simulink library "halin"  (R2021b)
settings: Solver=VariableStepAuto  StartTime=0.0  StopTime=10.0  RelTol=1e-3
undefined symbols (not defined in the file): TRUE
libraries: FVT_lib x100, hcu_lib x41
(part 7 of 10)

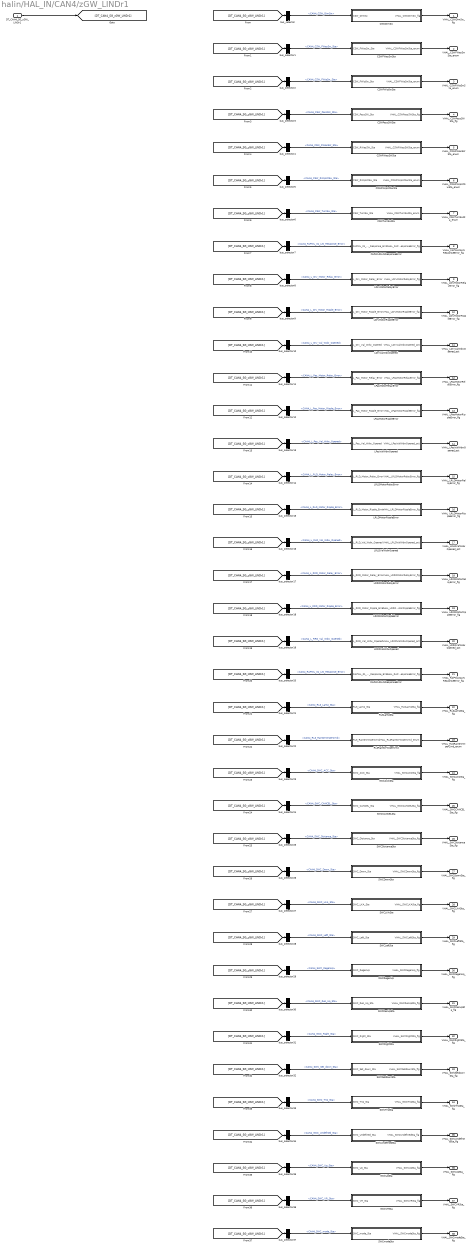
== system halin/HAL_IN/CAN4/zGW_LINDr1 ==
  DT_CAN4_SG_zGW_LINDr1 : Inport
  CSWDimSw : Subsystem
  CSWFWasSwSta : Subsystem
  CSWFWipSwSta : Subsystem
  CSWPassSWSta : Subsystem
  CSWRWasSWSta : Subsystem
  CSWRWipIntSwSta : Subsystem
  CSWTurnSwSta : Subsystem
  FAPWL01LINResponseError : Subsystem
  LDrvMotorRelayError : Subsystem
  LDrvMotorRippleError : Subsystem
  LDrvValWdwOpened : Subsystem
  LPasMotorRelayError : Subsystem
  LPasMotorRippleError : Subsystem
  LPasValWdwOpened : Subsystem
  LRLDMotorRelayError : Subsystem
  LRLDMotorRippleError : Subsystem
  LRLDValWdwOpened : Subsystem
  LRRDMotorRelayError : Subsystem
  LRRDMotorRippleError : Subsystem
  LRRDValWdwOpened : Subsystem
  RAPWL01LINResponseError : Subsystem
  RLSLampSta : Subsystem
  RLSRainSnrWiperCmd : Subsystem
  SWCACCSta : Subsystem
  SWCCANCELSta : Subsystem
  SWCDistanceSta : Subsystem
  SWCDownSta : Subsystem
  SWCLKASta : Subsystem
  SWCLeftSta : Subsystem
  SWCRegenUp : Subsystem
  SWCResUpSta : Subsystem
  SWCRightSta : Subsystem
  SWCSetdownSta : Subsystem
  SWCTripSta : Subsystem
  SWCUndefinedSta : Subsystem
  SWCUpSta : Subsystem
  SWCVRSta : Subsystem
  SWCmodeSta : Subsystem
  bus_selector : BusSelector  OutputSignals=CAN4_CSW_DimSw
  bus_selector1 : BusSelector  OutputSignals=CAN4_CSW_FWasSw_Sta
  bus_selector10 : BusSelector  OutputSignals=CAN4_L_Drv_Val_Wdw_Opened
  bus_selector11 : BusSelector  OutputSignals=CAN4_L_Pas_Motor_Relay_Error
  bus_selector12 : BusSelector  OutputSignals=CAN4_L_Pas_Motor_Ripple_Error
  bus_selector13 : BusSelector  OutputSignals=CAN4_L_Pas_Val_Wdw_Opened
  bus_selector14 : BusSelector  OutputSignals=CAN4_L_RLD_Motor_Relay_Error
  bus_selector15 : BusSelector  OutputSignals=CAN4_L_RLD_Motor_Ripple_Error
  bus_selector16 : BusSelector  OutputSignals=CAN4_L_RLD_Val_Wdw_Opened
  bus_selector17 : BusSelector  OutputSignals=CAN4_L_RRD_Motor_Relay_Error
  bus_selector18 : BusSelector  OutputSignals=CAN4_L_RRD_Motor_Ripple_Error
  bus_selector19 : BusSelector  OutputSignals=CAN4_L_RRD_Val_Wdw_Opened
  bus_selector2 : BusSelector  OutputSignals=CAN4_CSW_FWipSw_Sta
  bus_selector20 : BusSelector  OutputSignals=CAN4_RAPWL_01_LIN_Response_Error
  bus_selector21 : BusSelector  OutputSignals=CAN4_RLS_Lamp_Sta
  bus_selector22 : BusSelector  OutputSignals=CAN4_RLS_RainSnrWiperCmd
  bus_selector23 : BusSelector  OutputSignals=CAN4_SWC_ACC_Sta
  bus_selector24 : BusSelector  OutputSignals=CAN4_SWC_CANCEL_Sta
  bus_selector25 : BusSelector  OutputSignals=CAN4_SWC_Distance_Sta
  bus_selector26 : BusSelector  OutputSignals=CAN4_SWC_Down_Sta
  bus_selector27 : BusSelector  OutputSignals=CAN4_SWC_LKA_Sta
  bus_selector28 : BusSelector  OutputSignals=CAN4_SWC_Left_Sta
  bus_selector29 : BusSelector  OutputSignals=CAN4_SWC_RegenUp
  bus_selector3 : BusSelector  OutputSignals=CAN4_CSW_PassSW_Sta
  bus_selector30 : BusSelector  OutputSignals=CAN4_SWC_Res_Up_Sta
  bus_selector31 : BusSelector  OutputSignals=CAN4_SWC_Right_Sta
  bus_selector32 : BusSelector  OutputSignals=CAN4_SWC_Set_down_Sta
  bus_selector33 : BusSelector  OutputSignals=CAN4_SWC_Trip_Sta
  bus_selector34 : BusSelector  OutputSignals=CAN4_SWC_Undefined_Sta
  bus_selector35 : BusSelector  OutputSignals=CAN4_SWC_Up_Sta
  bus_selector36 : BusSelector  OutputSignals=CAN4_SWC_VR_Sta
  bus_selector37 : BusSelector  OutputSignals=CAN4_SWC_mode_Sta
  bus_selector4 : BusSelector  OutputSignals=CAN4_CSW_RWasSW_Sta
  bus_selector5 : BusSelector  OutputSignals=CAN4_CSW_RWipIntSw_Sta
  bus_selector6 : BusSelector  OutputSignals=CAN4_CSW_TurnSw_Sta
  bus_selector7 : BusSelector  OutputSignals=CAN4_FAPWL_01_LIN_Response_Error
  bus_selector8 : BusSelector  OutputSignals=CAN4_L_Drv_Motor_Relay_Error
  bus_selector9 : BusSelector  OutputSignals=CAN4_L_Drv_Motor_Ripple_Error
  VHAL_CSWDimSw_flg : Outport
  VHAL_CSWFWasSwSta_enum : Outport  Port=2
  VHAL_CSWFWipSwSta_enum : Outport  Port=3
  VHAL_CSWPassSWSta_flg : Outport  Port=4
  VHAL_CSWRWasSWSta_enum : Outport  Port=5
  VHAL_CSWRWipIntSwSta_enum : Outport  Port=6
  VHAL_CSWTurnSwSta_enum : Outport  Port=7
  VHAL_FAPWL01LINResponseError_flg : Outport  Port=8
  VHAL_LDrvMotorRelayError_flg : Outport  Port=9
  VHAL_LDrvMotorRippleError_flg : Outport  Port=10
  VHAL_LDrvValWdwOpened_pct : Outport  Port=11
  VHAL_LPasMotorRelayError_flg : Outport  Port=12
  VHAL_LPasMotorRippleError_flg : Outport  Port=13
  VHAL_LPasValWdwOpened_pct : Outport  Port=14
  VHAL_LRLDMotorRelayError_flg : Outport  Port=15
  VHAL_LRLDMotorRippleError_flg : Outport  Port=16
  VHAL_LRLDValWdwOpened_pct : Outport  Port=17
  VHAL_LRRDMotorRelayError_flg : Outport  Port=18
  VHAL_LRRDMotorRippleError_flg : Outport  Port=19
  VHAL_LRRDValWdwOpened_pct : Outport  Port=20
  VHAL_RAPWL01LINResponseError_flg : Outport  Port=21
  VHAL_RLSLampSta_flg : Outport  Port=22
  VHAL_RLSRainSnrWiperCmd_enum : Outport  Port=23
  VHAL_SWCACCSta_flg : Outport  Port=24
  VHAL_SWCCANCELSta_flg : Outport  Port=25
  VHAL_SWCDistanceSta_flg : Outport  Port=26
  VHAL_SWCDownSta_flg : Outport  Port=27
  VHAL_SWCLKASta_flg : Outport  Port=28
  VHAL_SWCLeftSta_flg : Outport  Port=29
  VHAL_SWCRegenUp_flg : Outport  Port=30
  VHAL_SWCResUpSta_flg : Outport  Port=31
  VHAL_SWCRightSta_flg : Outport  Port=32
  VHAL_SWCSetdownSta_flg : Outport  Port=33
  VHAL_SWCTripSta_flg : Outport  Port=34
  VHAL_SWCUndefinedSta_flg : Outport  Port=35
  VHAL_SWCUpSta_flg : Outport  Port=36
  VHAL_SWCVRSta_flg : Outport  Port=37
  VHAL_SWCmodeSta_flg : Outport  Port=38
  wires:
  DT_CAN4_SG_zGW_LINDr1/1 -> [DT_CAN4_SG_zGW_LINDr1]
  [DT_CAN4_SG_zGW_LINDr1] -> bus_selector/1
  bus_selector/1 -> CSWDimSw/1(CSW_DimSw)  "<CAN4_CSW_DimSw>"
  CSWDimSw/1(VHAL_CSWDimSw_flg) -> VHAL_CSWDimSw_flg/1
  [DT_CAN4_SG_zGW_LINDr1] -> bus_selector1/1
  bus_selector1/1 -> CSWFWasSwSta/1(CSW_FWasSw_Sta)  "<CAN4_CSW_FWasSw_Sta>"
  CSWFWasSwSta/1(VHAL_CSWFWasSwSta_enum) -> VHAL_CSWFWasSwSta_enum/1
  [DT_CAN4_SG_zGW_LINDr1] -> bus_selector2/1
  bus_selector2/1 -> CSWFWipSwSta/1(CSW_FWipSw_Sta)  "<CAN4_CSW_FWipSw_Sta>"
  CSWFWipSwSta/1(VHAL_CSWFWipSwSta_enum) -> VHAL_CSWFWipSwSta_enum/1
  [DT_CAN4_SG_zGW_LINDr1] -> bus_selector3/1
  bus_selector3/1 -> CSWPassSWSta/1(CSW_PassSW_Sta)  "<CAN4_CSW_PassSW_Sta>"
  CSWPassSWSta/1(VHAL_CSWPassSWSta_flg) -> VHAL_CSWPassSWSta_flg/1
  [DT_CAN4_SG_zGW_LINDr1] -> bus_selector4/1
  bus_selector4/1 -> CSWRWasSWSta/1(CSW_RWasSW_Sta)  "<CAN4_CSW_RWasSW_Sta>"
  CSWRWasSWSta/1(VHAL_CSWRWasSWSta_enum) -> VHAL_CSWRWasSWSta_enum/1
  [DT_CAN4_SG_zGW_LINDr1] -> bus_selector5/1
  bus_selector5/1 -> CSWRWipIntSwSta/1(CSW_RWipIntSw_Sta)  "<CAN4_CSW_RWipIntSw_Sta>"
  CSWRWipIntSwSta/1(VHAL_CSWRWipIntSwSta_enum) -> VHAL_CSWRWipIntSwSta_enum/1
  [DT_CAN4_SG_zGW_LINDr1] -> bus_selector6/1
  bus_selector6/1 -> CSWTurnSwSta/1(CSW_TurnSw_Sta)  "<CAN4_CSW_TurnSw_Sta>"
  CSWTurnSwSta/1(VHAL_CSWTurnSwSta_enum) -> VHAL_CSWTurnSwSta_enum/1
  [DT_CAN4_SG_zGW_LINDr1] -> bus_selector7/1
  bus_selector7/1 -> FAPWL01LINResponseError/1(FAPWL_01_LIN_Response_Error)  "<CAN4_FAPWL_01_LIN_Response_Error>"
  FAPWL01LINResponseError/1(VHAL_FAPWL01LINResponseError_flg) -> VHAL_FAPWL01LINResponseError_flg/1
  [DT_CAN4_SG_zGW_LINDr1] -> bus_selector8/1
  bus_selector8/1 -> LDrvMotorRelayError/1(L_Drv_Motor_Relay_Error)  "<CAN4_L_Drv_Motor_Relay_Error>"
  LDrvMotorRelayError/1(VHAL_LDrvMotorRelayError_flg) -> VHAL_LDrvMotorRelayError_flg/1
  [DT_CAN4_SG_zGW_LINDr1] -> bus_selector9/1
  bus_selector9/1 -> LDrvMotorRippleError/1(L_Drv_Motor_Ripple_Error)  "<CAN4_L_Drv_Motor_Ripple_Error>"
  LDrvMotorRippleError/1(VHAL_LDrvMotorRippleError_flg) -> VHAL_LDrvMotorRippleError_flg/1
  [DT_CAN4_SG_zGW_LINDr1] -> bus_selector10/1
  bus_selector10/1 -> LDrvValWdwOpened/1(L_Drv_Val_Wdw_Opened)  "<CAN4_L_Drv_Val_Wdw_Opened>"
  LDrvValWdwOpened/1(VHAL_LDrvValWdwOpened_pct) -> VHAL_LDrvValWdwOpened_pct/1
  [DT_CAN4_SG_zGW_LINDr1] -> bus_selector11/1
  bus_selector11/1 -> LPasMotorRelayError/1(L_Pas_Motor_Relay_Error)  "<CAN4_L_Pas_Motor_Relay_Error>"
  LPasMotorRelayError/1(VHAL_LPasMotorRelayError_flg) -> VHAL_LPasMotorRelayError_flg/1
  [DT_CAN4_SG_zGW_LINDr1] -> bus_selector12/1
  bus_selector12/1 -> LPasMotorRippleError/1(L_Pas_Motor_Ripple_Error)  "<CAN4_L_Pas_Motor_Ripple_Error>"
  LPasMotorRippleError/1(VHAL_LPasMotorRippleError_flg) -> VHAL_LPasMotorRippleError_flg/1
  [DT_CAN4_SG_zGW_LINDr1] -> bus_selector13/1
  bus_selector13/1 -> LPasValWdwOpened/1(L_Pas_Val_Wdw_Opened)  "<CAN4_L_Pas_Val_Wdw_Opened>"
  LPasValWdwOpened/1(VHAL_LPasValWdwOpened_pct) -> VHAL_LPasValWdwOpened_pct/1
  [DT_CAN4_SG_zGW_LINDr1] -> bus_selector14/1
  bus_selector14/1 -> LRLDMotorRelayError/1(L_RLD_Motor_Relay_Error)  "<CAN4_L_RLD_Motor_Relay_Error>"
  LRLDMotorRelayError/1(VHAL_LRLDMotorRelayError_flg) -> VHAL_LRLDMotorRelayError_flg/1
  [DT_CAN4_SG_zGW_LINDr1] -> bus_selector15/1
  bus_selector15/1 -> LRLDMotorRippleError/1(L_RLD_Motor_Ripple_Error)  "<CAN4_L_RLD_Motor_Ripple_Error>"
  LRLDMotorRippleError/1(VHAL_LRLDMotorRippleError_flg) -> VHAL_LRLDMotorRippleError_flg/1
  [DT_CAN4_SG_zGW_LINDr1] -> bus_selector16/1
  bus_selector16/1 -> LRLDValWdwOpened/1(L_RLD_Val_Wdw_Opened)  "<CAN4_L_RLD_Val_Wdw_Opened>"
  LRLDValWdwOpened/1(VHAL_LRLDValWdwOpened_pct) -> VHAL_LRLDValWdwOpened_pct/1
  [DT_CAN4_SG_zGW_LINDr1] -> bus_selector17/1
  bus_selector17/1 -> LRRDMotorRelayError/1(L_RRD_Motor_Relay_Error)  "<CAN4_L_RRD_Motor_Relay_Error>"
  LRRDMotorRelayError/1(VHAL_LRRDMotorRelayError_flg) -> VHAL_LRRDMotorRelayError_flg/1
  [DT_CAN4_SG_zGW_LINDr1] -> bus_selector18/1
  bus_selector18/1 -> LRRDMotorRippleError/1(L_RRD_Motor_Ripple_Error)  "<CAN4_L_RRD_Motor_Ripple_Error>"
  LRRDMotorRippleError/1(VHAL_LRRDMotorRippleError_flg) -> VHAL_LRRDMotorRippleError_flg/1
  [DT_CAN4_SG_zGW_LINDr1] -> bus_selector19/1
  bus_selector19/1 -> LRRDValWdwOpened/1(L_RRD_Val_Wdw_Opened)  "<CAN4_L_RRD_Val_Wdw_Opened>"
  LRRDValWdwOpened/1(VHAL_LRRDValWdwOpened_pct) -> VHAL_LRRDValWdwOpened_pct/1
  [DT_CAN4_SG_zGW_LINDr1] -> bus_selector20/1
  bus_selector20/1 -> RAPWL01LINResponseError/1(RAPWL_01_LIN_Response_Error)  "<CAN4_RAPWL_01_LIN_Response_Error>"
  RAPWL01LINResponseError/1(VHAL_RAPWL01LINResponseError_flg) -> VHAL_RAPWL01LINResponseError_flg/1
  [DT_CAN4_SG_zGW_LINDr1] -> bus_selector21/1
  bus_selector21/1 -> RLSLampSta/1(RLS_Lamp_Sta)  "<CAN4_RLS_Lamp_Sta>"
  RLSLampSta/1(VHAL_RLSLampSta_flg) -> VHAL_RLSLampSta_flg/1
  [DT_CAN4_SG_zGW_LINDr1] -> bus_selector22/1
  bus_selector22/1 -> RLSRainSnrWiperCmd/1(RLS_RainSnrWiperCmd)  "<CAN4_RLS_RainSnrWiperCmd>"
  RLSRainSnrWiperCmd/1(VHAL_RLSRainSnrWiperCmd_enum) -> VHAL_RLSRainSnrWiperCmd_enum/1
  [DT_CAN4_SG_zGW_LINDr1] -> bus_selector23/1
  bus_selector23/1 -> SWCACCSta/1(SWC_ACC_Sta)  "<CAN4_SWC_ACC_Sta>"
  SWCACCSta/1(VHAL_SWCACCSta_flg) -> VHAL_SWCACCSta_flg/1
  [DT_CAN4_SG_zGW_LINDr1] -> bus_selector24/1
  bus_selector24/1 -> SWCCANCELSta/1(SWC_CANCEL_Sta)  "<CAN4_SWC_CANCEL_Sta>"
  SWCCANCELSta/1(VHAL_SWCCANCELSta_flg) -> VHAL_SWCCANCELSta_flg/1
  [DT_CAN4_SG_zGW_LINDr1] -> bus_selector25/1
  bus_selector25/1 -> SWCDistanceSta/1(SWC_Distance_Sta)  "<CAN4_SWC_Distance_Sta>"
  SWCDistanceSta/1(VHAL_SWCDistanceSta_flg) -> VHAL_SWCDistanceSta_flg/1
  [DT_CAN4_SG_zGW_LINDr1] -> bus_selector26/1
  bus_selector26/1 -> SWCDownSta/1(SWC_Down_Sta)  "<CAN4_SWC_Down_Sta>"
  SWCDownSta/1(VHAL_SWCDownSta_flg) -> VHAL_SWCDownSta_flg/1
  [DT_CAN4_SG_zGW_LINDr1] -> bus_selector27/1
  bus_selector27/1 -> SWCLKASta/1(SWC_LKA_Sta)  "<CAN4_SWC_LKA_Sta>"
  SWCLKASta/1(VHAL_SWCLKASta_flg) -> VHAL_SWCLKASta_flg/1
  [DT_CAN4_SG_zGW_LINDr1] -> bus_selector28/1
  bus_selector28/1 -> SWCLeftSta/1(SWC_Left_Sta)  "<CAN4_SWC_Left_Sta>"
  SWCLeftSta/1(VHAL_SWCLeftSta_flg) -> VHAL_SWCLeftSta_flg/1
  [DT_CAN4_SG_zGW_LINDr1] -> bus_selector29/1
  bus_selector29/1 -> SWCRegenUp/1(SWC_RegenUp)  "<CAN4_SWC_RegenUp>"
  SWCRegenUp/1(VHAL_SWCRegenUp_flg) -> VHAL_SWCRegenUp_flg/1
  [DT_CAN4_SG_zGW_LINDr1] -> bus_selector30/1
  bus_selector30/1 -> SWCResUpSta/1(SWC_Res_Up_Sta)  "<CAN4_SWC_Res_Up_Sta>"
  SWCResUpSta/1(VHAL_SWCResUpSta_flg) -> VHAL_SWCResUpSta_flg/1
  [DT_CAN4_SG_zGW_LINDr1] -> bus_selector31/1
  bus_selector31/1 -> SWCRightSta/1(SWC_Right_Sta)  "<CAN4_SWC_Right_Sta>"
  SWCRightSta/1(VHAL_SWCRightSta_flg) -> VHAL_SWCRightSta_flg/1
  [DT_CAN4_SG_zGW_LINDr1] -> bus_selector32/1
  bus_selector32/1 -> SWCSetdownSta/1(SWC_Set_down_Sta)  "<CAN4_SWC_Set_down_Sta>"
  SWCSetdownSta/1(VHAL_SWCSetdownSta_flg) -> VHAL_SWCSetdownSta_flg/1
  [DT_CAN4_SG_zGW_LINDr1] -> bus_selector33/1
  bus_selector33/1 -> SWCTripSta/1(SWC_Trip_Sta)  "<CAN4_SWC_Trip_Sta>"
  SWCTripSta/1(VHAL_SWCTripSta_flg) -> VHAL_SWCTripSta_flg/1
  [DT_CAN4_SG_zGW_LINDr1] -> bus_selector34/1
  bus_selector34/1 -> SWCUndefinedSta/1(SWC_Undefined_Sta)  "<CAN4_SWC_Undefined_Sta>"
  SWCUndefinedSta/1(VHAL_SWCUndefinedSta_flg) -> VHAL_SWCUndefinedSta_flg/1
  [DT_CAN4_SG_zGW_LINDr1] -> bus_selector35/1
  bus_selector35/1 -> SWCUpSta/1(SWC_Up_Sta)  "<CAN4_SWC_Up_Sta>"
  SWCUpSta/1(VHAL_SWCUpSta_flg) -> VHAL_SWCUpSta_flg/1
  [DT_CAN4_SG_zGW_LINDr1] -> bus_selector36/1
  bus_selector36/1 -> SWCVRSta/1(SWC_VR_Sta)  "<CAN4_SWC_VR_Sta>"
  SWCVRSta/1(VHAL_SWCVRSta_flg) -> VHAL_SWCVRSta_flg/1
  [DT_CAN4_SG_zGW_LINDr1] -> bus_selector37/1
  bus_selector37/1 -> SWCmodeSta/1(SWC_mode_Sta)  "<CAN4_SWC_mode_Sta>"
  SWCmodeSta/1(VHAL_SWCmodeSta_flg) -> VHAL_SWCmodeSta_flg/1

== system halin/HAL_IN/CAN5/TBOX1 ==
  DT_CAN5_SG_TBOX1 : Inport
  CbnPreACEnaReq : Subsystem
  PowerOffTSet : Subsystem
  ReDoorLock : Subsystem
  ReOutsideMirror : Subsystem
  RePwrReqTbox : Subsystem
  ReRadio : Subsystem
  RemoteACTemp : Subsystem
  RemoteAutoReq : Subsystem
  TBOXNETSIGSTR : Subsystem
  TBOXTESTSTATUS : Subsystem
  bus_selector : BusSelector  OutputSignals=CAN5_CbnPreACEnaReq
  bus_selector1 : BusSelector  OutputSignals=CAN5_PowerOff_T_Set
  bus_selector2 : BusSelector  OutputSignals=CAN5_ReOutsideMirror
  bus_selector3 : BusSelector  OutputSignals=CAN5_Re_DoorLock
  bus_selector4 : BusSelector  OutputSignals=CAN5_Re_PwrReqTbox
  bus_selector5 : BusSelector  OutputSignals=CAN5_Re_Radio
  bus_selector6 : BusSelector  OutputSignals=CAN5_Remote_ACTemp
  bus_selector7 : BusSelector  OutputSignals=CAN5_Remote_AutoReq
  bus_selector8 : BusSelector  OutputSignals=CAN5_TBOX_NET_SIG_STR
  bus_selector9 : BusSelector  OutputSignals=CAN5_TBOX_TEST_STATUS
  VHAL_CbnPreACEnaReq_enum : Outport
  VHAL_PowerOffTSet_cnt : Outport  Port=2
  VHAL_ReOutsideMirror_enum : Outport  Port=3
  VHAL_ReDoorLock_enum : Outport  Port=4
  VHAL_RePwrReqTbox_enum : Outport  Port=5
  VHAL_ReRadio_flg : Outport  Port=6
  VHAL_RemoteACTemp_C : Outport  Port=7
  VHAL_RemoteAutoReq_flg : Outport  Port=8
  VHAL_TBOXNETSIGSTR_enum : Outport  Port=9
  VHAL_TBOXTESTSTATUS_enum : Outport  Port=10
  wires:
  DT_CAN5_SG_TBOX1/1 -> [DT_CAN5_SG_TBOX1]
  [DT_CAN5_SG_TBOX1] -> bus_selector/1
  bus_selector/1 -> CbnPreACEnaReq/1(CbnPreACEnaReq)  "<CAN5_CbnPreACEnaReq>"
  CbnPreACEnaReq/1(VHAL_CbnPreACEnaReq_enum) -> VHAL_CbnPreACEnaReq_enum/1
  [DT_CAN5_SG_TBOX1] -> bus_selector1/1
  bus_selector1/1 -> PowerOffTSet/1(PowerOff_T_Set)  "<CAN5_PowerOff_T_Set>"
  PowerOffTSet/1(VHAL_PowerOffTSet_cnt) -> VHAL_PowerOffTSet_cnt/1
  [DT_CAN5_SG_TBOX1] -> bus_selector2/1
  bus_selector2/1 -> ReOutsideMirror/1(ReOutsideMirror)  "<CAN5_ReOutsideMirror>"
  ReOutsideMirror/1(VHAL_ReOutsideMirror_enum) -> VHAL_ReOutsideMirror_enum/1
  [DT_CAN5_SG_TBOX1] -> bus_selector3/1
  bus_selector3/1 -> ReDoorLock/1(Re_DoorLock)  "<CAN5_Re_DoorLock>"
  ReDoorLock/1(VHAL_ReDoorLock_enum) -> VHAL_ReDoorLock_enum/1
  [DT_CAN5_SG_TBOX1] -> bus_selector4/1
  bus_selector4/1 -> RePwrReqTbox/1(Re_PwrReqTbox)  "<CAN5_Re_PwrReqTbox>"
  RePwrReqTbox/1(VHAL_RePwrReqTbox_enum) -> VHAL_RePwrReqTbox_enum/1
  [DT_CAN5_SG_TBOX1] -> bus_selector5/1
  bus_selector5/1 -> ReRadio/1(Re_Radio)  "<CAN5_Re_Radio>"
  ReRadio/1(VHAL_ReRadio_flg) -> VHAL_ReRadio_flg/1
  [DT_CAN5_SG_TBOX1] -> bus_selector6/1
  bus_selector6/1 -> RemoteACTemp/1(Remote_ACTemp)  "<CAN5_Remote_ACTemp>"
  RemoteACTemp/1(VHAL_RemoteACTemp_C) -> VHAL_RemoteACTemp_C/1
  [DT_CAN5_SG_TBOX1] -> bus_selector7/1
  bus_selector7/1 -> RemoteAutoReq/1(Remote_AutoReq)  "<CAN5_Remote_AutoReq>"
  RemoteAutoReq/1(VHAL_RemoteAutoReq_flg) -> VHAL_RemoteAutoReq_flg/1
  [DT_CAN5_SG_TBOX1] -> bus_selector8/1
  bus_selector8/1 -> TBOXNETSIGSTR/1(TBOX_NET_SIG_STR)  "<CAN5_TBOX_NET_SIG_STR>"
  TBOXNETSIGSTR/1(VHAL_TBOXNETSIGSTR_enum) -> VHAL_TBOXNETSIGSTR_enum/1
  [DT_CAN5_SG_TBOX1] -> bus_selector9/1
  bus_selector9/1 -> TBOXTESTSTATUS/1(TBOX_TEST_STATUS)  "<CAN5_TBOX_TEST_STATUS>"
  TBOXTESTSTATUS/1(VHAL_TBOXTESTSTATUS_enum) -> VHAL_TBOXTESTSTATUS_enum/1

== system halin/HAL_IN/CAN5/TBOX2 ==
  DT_CAN5_SG_TBOX2 : Inport
  TimeSyncFromBSDay : Subsystem
  TimeSyncFromBSHour : Subsystem
  TimeSyncFromBSMinute : Subsystem
  TimeSyncFromBSMonth : Subsystem
  TimeSyncFromBSSecond : Subsystem
  TimeSyncFromBSYear : Subsystem
  bus_selector : BusSelector  OutputSignals=CAN5_TimeSyncFromBS_Day
  bus_selector1 : BusSelector  OutputSignals=CAN5_TimeSyncFromBS_Hour
  bus_selector2 : BusSelector  OutputSignals=CAN5_TimeSyncFromBS_Minute
  bus_selector3 : BusSelector  OutputSignals=CAN5_TimeSyncFromBS_Month
  bus_selector4 : BusSelector  OutputSignals=CAN5_TimeSyncFromBS_Second
  bus_selector5 : BusSelector  OutputSignals=CAN5_TimeSyncFromBS_Year
  VHAL_TimeSyncFromBSDay_DAY : Outport
  VHAL_TimeSyncFromBSHour_hr : Outport  Port=2
  VHAL_TimeSyncFromBSMinute_min : Outport  Port=3
  VHAL_TimeSyncFromBSMonth_MONTH : Outport  Port=4
  VHAL_TimeSyncFromBSSecond_s : Outport  Port=5
  VHAL_TimeSyncFromBSYear_YEAR : Outport  Port=6
  wires:
  DT_CAN5_SG_TBOX2/1 -> [DT_CAN5_SG_TBOX2]
  [DT_CAN5_SG_TBOX2] -> bus_selector/1
  bus_selector/1 -> TimeSyncFromBSDay/1(TimeSyncFromBS_Day)  "<CAN5_TimeSyncFromBS_Day>"
  TimeSyncFromBSDay/1(VHAL_TimeSyncFromBSDay_DAY) -> VHAL_TimeSyncFromBSDay_DAY/1
  [DT_CAN5_SG_TBOX2] -> bus_selector1/1
  bus_selector1/1 -> TimeSyncFromBSHour/1(TimeSyncFromBS_Hour)  "<CAN5_TimeSyncFromBS_Hour>"
  TimeSyncFromBSHour/1(VHAL_TimeSyncFromBSHour_hr) -> VHAL_TimeSyncFromBSHour_hr/1
  [DT_CAN5_SG_TBOX2] -> bus_selector2/1
  bus_selector2/1 -> TimeSyncFromBSMinute/1(TimeSyncFromBS_Minute)  "<CAN5_TimeSyncFromBS_Minute>"
  TimeSyncFromBSMinute/1(VHAL_TimeSyncFromBSMinute_min) -> VHAL_TimeSyncFromBSMinute_min/1
  [DT_CAN5_SG_TBOX2] -> bus_selector3/1
  bus_selector3/1 -> TimeSyncFromBSMonth/1(TimeSyncFromBS_Month)  "<CAN5_TimeSyncFromBS_Month>"
  TimeSyncFromBSMonth/1(VHAL_TimeSyncFromBSMonth_MONTH) -> VHAL_TimeSyncFromBSMonth_MONTH/1
  [DT_CAN5_SG_TBOX2] -> bus_selector4/1
  bus_selector4/1 -> TimeSyncFromBSSecond/1(TimeSyncFromBS_Second)  "<CAN5_TimeSyncFromBS_Second>"
  TimeSyncFromBSSecond/1(VHAL_TimeSyncFromBSSecond_s) -> VHAL_TimeSyncFromBSSecond_s/1
  [DT_CAN5_SG_TBOX2] -> bus_selector5/1
  bus_selector5/1 -> TimeSyncFromBSYear/1(TimeSyncFromBS_Year)  "<CAN5_TimeSyncFromBS_Year>"
  TimeSyncFromBSYear/1(VHAL_TimeSyncFromBSYear_YEAR) -> VHAL_TimeSyncFromBSYear_YEAR/1

== system halin/HAL_IN/CAN5/TBOX3 ==
  DT_CAN5_SG_TBOX3 : Inport
  ChargePercentSet : Subsystem
  ReserveChargeOFFDay : Subsystem
  ReserveChargeOFFHour : Subsystem
  ReserveChargeOFFMinute : Subsystem
  ReserveChargeOFFMonth : Subsystem
  ReserveChargeOFFYear : Subsystem
  ReserveChargeOnDay : Subsystem
  ReserveChargeOnHour : Subsystem
  ReserveChargeOnMinute : Subsystem
  ReserveChargeOnMonth : Subsystem
  ReserveChargeOnYear : Subsystem
  TBOXHWVER : Subsystem
  TBOXSWVER : Subsystem
  bus_selector : BusSelector  OutputSignals=CAN5_Charge_Percent_Set
  bus_selector1 : BusSelector  OutputSignals=CAN5_ReserveChargeOFF_Day
  bus_selector10 : BusSelector  OutputSignals=CAN5_ReserveChargeOn_Year
  bus_selector11 : BusSelector  OutputSignals=CAN5_TBOX_HW_VER
  bus_selector12 : BusSelector  OutputSignals=CAN5_TBOX_SW_VER
  bus_selector2 : BusSelector  OutputSignals=CAN5_ReserveChargeOFF_Hour
  bus_selector3 : BusSelector  OutputSignals=CAN5_ReserveChargeOFF_Minute
  bus_selector4 : BusSelector  OutputSignals=CAN5_ReserveChargeOFF_Month
  bus_selector5 : BusSelector  OutputSignals=CAN5_ReserveChargeOFF_Year
  bus_selector6 : BusSelector  OutputSignals=CAN5_ReserveChargeOn_Day
  bus_selector7 : BusSelector  OutputSignals=CAN5_ReserveChargeOn_Hour
  bus_selector8 : BusSelector  OutputSignals=CAN5_ReserveChargeOn_Minute
  bus_selector9 : BusSelector  OutputSignals=CAN5_ReserveChargeOn_Month
  VHAL_ChargePercentSet_pct : Outport
  VHAL_ReserveChargeOFFDay_DAY : Outport  Port=2
  VHAL_ReserveChargeOFFHour_hr : Outport  Port=3
  VHAL_ReserveChargeOFFMinute_min : Outport  Port=4
  VHAL_ReserveChargeOFFMonth_MONTH : Outport  Port=5
  VHAL_ReserveChargeOFFYear_YEAR : Outport  Port=6
  VHAL_ReserveChargeOnDay_DAY : Outport  Port=7
  VHAL_ReserveChargeOnHour_hr : Outport  Port=8
  VHAL_ReserveChargeOnMinute_min : Outport  Port=9
  VHAL_ReserveChargeOnMonth_MONTH : Outport  Port=10
  VHAL_ReserveChargeOnYear_YEAR : Outport  Port=11
  VHAL_TBOXHWVER_enum : Outport  Port=12
  VHAL_TBOXSWVER_enum : Outport  Port=13
  wires:
  DT_CAN5_SG_TBOX3/1 -> [DT_CAN5_SG_TBOX3]
  [DT_CAN5_SG_TBOX3] -> bus_selector/1
  bus_selector/1 -> ChargePercentSet/1(Charge_Percent_Set)  "<CAN5_Charge_Percent_Set>"
  ChargePercentSet/1(VHAL_ChargePercentSet_pct) -> VHAL_ChargePercentSet_pct/1
  [DT_CAN5_SG_TBOX3] -> bus_selector1/1
  bus_selector1/1 -> ReserveChargeOFFDay/1(ReserveChargeOFF_Day)  "<CAN5_ReserveChargeOFF_Day>"
  ReserveChargeOFFDay/1(VHAL_ReserveChargeOFFDay_DAY) -> VHAL_ReserveChargeOFFDay_DAY/1
  [DT_CAN5_SG_TBOX3] -> bus_selector2/1
  bus_selector2/1 -> ReserveChargeOFFHour/1(ReserveChargeOFF_Hour)  "<CAN5_ReserveChargeOFF_Hour>"
  ReserveChargeOFFHour/1(VHAL_ReserveChargeOFFHour_hr) -> VHAL_ReserveChargeOFFHour_hr/1
  [DT_CAN5_SG_TBOX3] -> bus_selector3/1
  bus_selector3/1 -> ReserveChargeOFFMinute/1(ReserveChargeOFF_Minute)  "<CAN5_ReserveChargeOFF_Minute>"
  ReserveChargeOFFMinute/1(VHAL_ReserveChargeOFFMinute_min) -> VHAL_ReserveChargeOFFMinute_min/1
  [DT_CAN5_SG_TBOX3] -> bus_selector4/1
  bus_selector4/1 -> ReserveChargeOFFMonth/1(ReserveChargeOFF_Month)  "<CAN5_ReserveChargeOFF_Month>"
  ReserveChargeOFFMonth/1(VHAL_ReserveChargeOFFMonth_MONTH) -> VHAL_ReserveChargeOFFMonth_MONTH/1
  [DT_CAN5_SG_TBOX3] -> bus_selector5/1
  bus_selector5/1 -> ReserveChargeOFFYear/1(ReserveChargeOFF_Year)  "<CAN5_ReserveChargeOFF_Year>"
  ReserveChargeOFFYear/1(VHAL_ReserveChargeOFFYear_YEAR) -> VHAL_ReserveChargeOFFYear_YEAR/1
  [DT_CAN5_SG_TBOX3] -> bus_selector6/1
  bus_selector6/1 -> ReserveChargeOnDay/1(ReserveChargeOn_Day)  "<CAN5_ReserveChargeOn_Day>"
  ReserveChargeOnDay/1(VHAL_ReserveChargeOnDay_DAY) -> VHAL_ReserveChargeOnDay_DAY/1
  [DT_CAN5_SG_TBOX3] -> bus_selector7/1
  bus_selector7/1 -> ReserveChargeOnHour/1(ReserveChargeOn_Hour)  "<CAN5_ReserveChargeOn_Hour>"
  ReserveChargeOnHour/1(VHAL_ReserveChargeOnHour_hr) -> VHAL_ReserveChargeOnHour_hr/1
  [DT_CAN5_SG_TBOX3] -> bus_selector8/1
  bus_selector8/1 -> ReserveChargeOnMinute/1(ReserveChargeOn_Minute)  "<CAN5_ReserveChargeOn_Minute>"
  ReserveChargeOnMinute/1(VHAL_ReserveChargeOnMinute_min) -> VHAL_ReserveChargeOnMinute_min/1
  [DT_CAN5_SG_TBOX3] -> bus_selector9/1
  bus_selector9/1 -> ReserveChargeOnMonth/1(ReserveChargeOn_Month)  "<CAN5_ReserveChargeOn_Month>"
  ReserveChargeOnMonth/1(VHAL_ReserveChargeOnMonth_MONTH) -> VHAL_ReserveChargeOnMonth_MONTH/1
  [DT_CAN5_SG_TBOX3] -> bus_selector10/1
  bus_selector10/1 -> ReserveChargeOnYear/1(ReserveChargeOn_Year)  "<CAN5_ReserveChargeOn_Year>"
  ReserveChargeOnYear/1(VHAL_ReserveChargeOnYear_YEAR) -> VHAL_ReserveChargeOnYear_YEAR/1
  [DT_CAN5_SG_TBOX3] -> bus_selector11/1
  bus_selector11/1 -> TBOXHWVER/1(TBOX_HW_VER)  "<CAN5_TBOX_HW_VER>"
  TBOXHWVER/1(VHAL_TBOXHWVER_enum) -> VHAL_TBOXHWVER_enum/1
  [DT_CAN5_SG_TBOX3] -> bus_selector12/1
  bus_selector12/1 -> TBOXSWVER/1(TBOX_SW_VER)  "<CAN5_TBOX_SW_VER>"
  TBOXSWVER/1(VHAL_TBOXSWVER_enum) -> VHAL_TBOXSWVER_enum/1

== system halin/HAL_IN/CAN5/VHAL_CANMsgInvalidTBOX1_flg ==
  Cast To Boolean13 : DataTypeConversion  OutDataTypeStr=boolean
  Constant : Constant  Value=TRUE
  Latch13 : hcu_lib/Basic_Blocks/Latch
  Switch13 : Switch  Criteria=u2 ~= 0
  Unit Delay : UnitDelay  SampleTime=-1  HasFrameUpgradeWarning=on
  UnitConverter : DataTypeConversion  OutDataTypeStr=boolean
  Out : Outport
  wires:
  Constant/1 -> Switch13/3
  Unit Delay/1 -> Cast To Boolean13/1
  Cast To Boolean13/1 -> Switch13/1, Latch13/1
  Switch13/1 -> UnitConverter/1
  Latch13/1 -> Switch13/2
  UnitConverter/1 -> Unit Delay/1, Out/1  "VHAL_CANMsgInvalidTBOX1_flg"

== system halin/HAL_IN/CAN5/VHAL_CANMsgInvalidTBOX2_flg ==
  Cast To Boolean13 : DataTypeConversion  OutDataTypeStr=boolean
  Constant : Constant  Value=TRUE
  Latch13 : hcu_lib/Basic_Blocks/Latch
  Switch13 : Switch  Criteria=u2 ~= 0
  Unit Delay : UnitDelay  SampleTime=-1  HasFrameUpgradeWarning=on
  UnitConverter : DataTypeConversion  OutDataTypeStr=boolean
  Out : Outport
  wires:
  Constant/1 -> Switch13/3
  Unit Delay/1 -> Cast To Boolean13/1
  Cast To Boolean13/1 -> Switch13/1, Latch13/1
  Switch13/1 -> UnitConverter/1
  Latch13/1 -> Switch13/2
  UnitConverter/1 -> Unit Delay/1, Out/1  "VHAL_CANMsgInvalidTBOX2_flg"

== system halin/HAL_IN/CAN5/VHAL_CANMsgInvalidTBOX3_flg ==
  Cast To Boolean13 : DataTypeConversion  OutDataTypeStr=boolean
  Constant : Constant  Value=TRUE
  Latch13 : hcu_lib/Basic_Blocks/Latch
  Switch13 : Switch  Criteria=u2 ~= 0
  Unit Delay : UnitDelay  SampleTime=-1  HasFrameUpgradeWarning=on
  UnitConverter : DataTypeConversion  OutDataTypeStr=boolean
  Out : Outport
  wires:
  Constant/1 -> Switch13/3
  Unit Delay/1 -> Cast To Boolean13/1
  Cast To Boolean13/1 -> Switch13/1, Latch13/1
  Switch13/1 -> UnitConverter/1
  Latch13/1 -> Switch13/2
  UnitConverter/1 -> Unit Delay/1, Out/1  "VHAL_CANMsgInvalidTBOX3_flg"

== system halin/HAL_IN/CAN7/Door_Fr1 ==
  DT_CAN7_SG_Door_Fr1 : Inport
  DoorFrDoorEmergencysta : Subsystem
  DoorFrDooroperationsta : Subsystem
  DoorFrDoorpositionsta : Subsystem
  bus_selector : BusSelector  OutputSignals=CAN7_Door_Fr_DoorEmergency_sta
  bus_selector1 : BusSelector  OutputSignals=CAN7_Door_Fr_Dooroperation_sta
  bus_selector2 : BusSelector  OutputSignals=CAN7_Door_Fr_Doorposition_sta
  VHAL_DoorFrDoorEmergencysta_enum : Outport
  VHAL_DoorFrDooroperationsta_enum : Outport  Port=2
  VHAL_DoorFrDoorpositionsta_enum : Outport  Port=3
  wires:
  DT_CAN7_SG_Door_Fr1/1 -> [DT_CAN7_SG_Door_Fr1]
  [DT_CAN7_SG_Door_Fr1] -> bus_selector/1
  bus_selector/1 -> DoorFrDoorEmergencysta/1(Door_Fr_DoorEmergency_sta)  "<CAN7_Door_Fr_DoorEmergency_sta>"
  DoorFrDoorEmergencysta/1(VHAL_DoorFrDoorEmergencysta_enum) -> VHAL_DoorFrDoorEmergencysta_enum/1
  [DT_CAN7_SG_Door_Fr1] -> bus_selector1/1
  bus_selector1/1 -> DoorFrDooroperationsta/1(Door_Fr_Dooroperation_sta)  "<CAN7_Door_Fr_Dooroperation_sta>"
  DoorFrDooroperationsta/1(VHAL_DoorFrDooroperationsta_enum) -> VHAL_DoorFrDooroperationsta_enum/1
  [DT_CAN7_SG_Door_Fr1] -> bus_selector2/1
  bus_selector2/1 -> DoorFrDoorpositionsta/1(Door_Fr_Doorposition_sta)  "<CAN7_Door_Fr_Doorposition_sta>"
  DoorFrDoorpositionsta/1(VHAL_DoorFrDoorpositionsta_enum) -> VHAL_DoorFrDoorpositionsta_enum/1

== system halin/HAL_IN/CAN7/VHAL_CANMsgInvalidDoorFr1_flg ==
  Cast To Boolean13 : DataTypeConversion  OutDataTypeStr=boolean
  Constant : Constant  Value=TRUE
  Latch13 : hcu_lib/Basic_Blocks/Latch
  Switch13 : Switch  Criteria=u2 ~= 0
  Unit Delay : UnitDelay  SampleTime=-1  HasFrameUpgradeWarning=on
  UnitConverter : DataTypeConversion  OutDataTypeStr=boolean
  Out : Outport
  wires:
  Constant/1 -> Switch13/3
  Unit Delay/1 -> Cast To Boolean13/1
  Cast To Boolean13/1 -> Switch13/1, Latch13/1
  Switch13/1 -> UnitConverter/1
  Latch13/1 -> Switch13/2
  UnitConverter/1 -> Unit Delay/1, Out/1  "VHAL_CANMsgInvalidDoorFr1_flg"

== system halin/HAL_IN/CAN1/DCDC_Status_1/DCDCEnSta ==
  DCDCEnSta : Inport
  UnitConverter : DataTypeConversion  OutDataTypeStr=uint8
  VHAL_DCDCEnSta_enum : Outport
  wires:
  UnitConverter/1 -> VHAL_DCDCEnSta_enum/1
  DCDCEnSta/1 -> UnitConverter/1

== system halin/HAL_IN/CAN1/DCDC_Status_2/DCDCOutVol ==
  DCDCOutVol : Inport
  UnitConverter : DataTypeConversion  OutDataTypeStr=uint16
  convert_in : FVT_lib/hal/convert_in  gain=0.1  offset=0
  VHAL_DCDCOutVol_V : Outport
  wires:
  convert_in/1 -> VHAL_DCDCOutVol_V/1
  UnitConverter/1 -> convert_in/1
  DCDCOutVol/1 -> UnitConverter/1

== system halin/HAL_IN/CAN1/EAC_Status_1/EACEnSta ==
  EACEnSta : Inport
  UnitConverter : DataTypeConversion  OutDataTypeStr=uint8
  VHAL_EACEnSta_enum : Outport
  wires:
  UnitConverter/1 -> VHAL_EACEnSta_enum/1
  EACEnSta/1 -> UnitConverter/1

== system halin/HAL_IN/CAN1/EBC1/ABSFullyOper ==
  ABSFullyOper : Inport
  UnitConverter : DataTypeConversion  OutDataTypeStr=uint8
  VHAL_ABSFullyOper_enum : Outport
  wires:
  UnitConverter/1 -> VHAL_ABSFullyOper_enum/1
  ABSFullyOper/1 -> UnitConverter/1

== system halin/HAL_IN/CAN1/EBC1/ABSOffroadSw ==
  ABSOffroadSw : Inport
  UnitConverter : DataTypeConversion  OutDataTypeStr=uint8
  VHAL_ABSOffroadSw_enum : Outport
  wires:
  UnitConverter/1 -> VHAL_ABSOffroadSw_enum/1
  ABSOffroadSw/1 -> UnitConverter/1

== system halin/HAL_IN/CAN1/EBC1/ASRBrakeCtrlAtc ==
  ASRBrakeCtrlAtc : Inport
  UnitConverter : DataTypeConversion  OutDataTypeStr=uint8
  VHAL_ASRBrakeCtrlAtc_enum : Outport
  wires:
  UnitConverter/1 -> VHAL_ASRBrakeCtrlAtc_enum/1
  ASRBrakeCtrlAtc/1 -> UnitConverter/1

== system halin/HAL_IN/CAN1/EBC1/ASREngCtrlAtc ==
  ASREngCtrlAtc : Inport
  UnitConverter : DataTypeConversion  OutDataTypeStr=uint8
  VHAL_ASREngCtrlAtc_enum : Outport
  wires:
  UnitConverter/1 -> VHAL_ASREngCtrlAtc_enum/1
  ASREngCtrlAtc/1 -> UnitConverter/1

== system halin/HAL_IN/CAN1/EBC1/ASRHillHolderSw ==
  ASRHillHolderSw : Inport
  UnitConverter : DataTypeConversion  OutDataTypeStr=uint8
  VHAL_ASRHillHolderSw_enum : Outport
  wires:
  UnitConverter/1 -> VHAL_ASRHillHolderSw_enum/1
  ASRHillHolderSw/1 -> UnitConverter/1

== system halin/HAL_IN/CAN1/EBC1/ASROffroadSw ==
  ASROffroadSw : Inport
  UnitConverter : DataTypeConversion  OutDataTypeStr=uint8
  VHAL_ASROffroadSw_enum : Outport
  wires:
  UnitConverter/1 -> VHAL_ASROffroadSw_enum/1
  ASROffroadSw/1 -> UnitConverter/1

== system halin/HAL_IN/CAN1/EBC1/ATCASRInfoSig ==
  ATCASRInfoSig : Inport
  UnitConverter : DataTypeConversion  OutDataTypeStr=uint8
  VHAL_ATCASRInfoSig_enum : Outport
  wires:
  UnitConverter/1 -> VHAL_ATCASRInfoSig_enum/1
  ATCASRInfoSig/1 -> UnitConverter/1

== system halin/HAL_IN/CAN1/EBC1/AcltrInterlockSw ==
  AcltrInterlockSw : Inport
  UnitConverter : DataTypeConversion  OutDataTypeStr=uint8
  VHAL_AcltrInterlockSw_enum : Outport
  wires:
  UnitConverter/1 -> VHAL_AcltrInterlockSw_enum/1
  AcltrInterlockSw/1 -> UnitConverter/1

== system halin/HAL_IN/CAN1/EBC1/AntiLBrakABSAct ==
  AntiLBrakABSAct : Inport
  UnitConverter : DataTypeConversion  OutDataTypeStr=uint8
  VHAL_AntiLBrakABSAct_enum : Outport
  wires:
  UnitConverter/1 -> VHAL_AntiLBrakABSAct_enum/1
  AntiLBrakABSAct/1 -> UnitConverter/1

== system halin/HAL_IN/CAN1/EBC1/BrakePedalPos ==
  BrakePedalPos : Inport
  UnitConverter : DataTypeConversion  OutDataTypeStr=uint8
  convert_in : FVT_lib/hal/convert_in  gain=0.4  offset=0
  VHAL_BrakePedalPos_pct : Outport
  wires:
  convert_in/1 -> VHAL_BrakePedalPos_pct/1
  UnitConverter/1 -> convert_in/1
  BrakePedalPos/1 -> UnitConverter/1

== system halin/HAL_IN/CAN1/EBC1/EBSAmWarnLampSta ==
  EBSAmWarnLampSta : Inport
  UnitConverter : DataTypeConversion  OutDataTypeStr=uint8
  VHAL_EBSAmWarnLampSta_enum : Outport
  wires:
  UnitConverter/1 -> VHAL_EBSAmWarnLampSta_enum/1
  EBSAmWarnLampSta/1 -> UnitConverter/1

== system halin/HAL_IN/CAN1/EBC1/EBSBrakeSw ==
  EBSBrakeSw : Inport
  UnitConverter : DataTypeConversion  OutDataTypeStr=uint8
  VHAL_EBSBrakeSw_enum : Outport
  wires:
  UnitConverter/1 -> VHAL_EBSBrakeSw_enum/1
  EBSBrakeSw/1 -> UnitConverter/1

== system halin/HAL_IN/CAN1/EBC1/EBSRedWarnLampSta ==
  EBSRedWarnLampSta : Inport
  UnitConverter : DataTypeConversion  OutDataTypeStr=uint8
  VHAL_EBSRedWarnLampSta_enum : Outport
  wires:
  UnitConverter/1 -> VHAL_EBSRedWarnLampSta_enum/1
  EBSRedWarnLampSta/1 -> UnitConverter/1

== system halin/HAL_IN/CAN1/EBC1/EngAuxShutdownSw ==
  EngAuxShutdownSw : Inport
  UnitConverter : DataTypeConversion  OutDataTypeStr=uint8
  VHAL_EngAuxShutdownSw_enum : Outport
  wires:
  UnitConverter/1 -> VHAL_EngAuxShutdownSw_enum/1
  EngAuxShutdownSw/1 -> UnitConverter/1

== system halin/HAL_IN/CAN1/EBC1/EngDerateSw ==
  EngDerateSw : Inport
  UnitConverter : DataTypeConversion  OutDataTypeStr=uint8
  VHAL_EngDerateSw_enum : Outport
  wires:
  UnitConverter/1 -> VHAL_EngDerateSw_enum/1
  EngDerateSw/1 -> UnitConverter/1

== system halin/HAL_IN/CAN1/EBC1/EngRetSel ==
  EngRetSel : Inport
  UnitConverter : DataTypeConversion  OutDataTypeStr=uint8
  convert_in : FVT_lib/hal/convert_in  gain=0.4  offset=0
  VHAL_EngRetSel_pct : Outport
  wires:
  convert_in/1 -> VHAL_EngRetSel_pct/1
  UnitConverter/1 -> convert_in/1
  EngRetSel/1 -> UnitConverter/1

== system halin/HAL_IN/CAN1/EBC1/HaltBrakeSw ==
  HaltBrakeSw : Inport
  UnitConverter : DataTypeConversion  OutDataTypeStr=uint8
  VHAL_HaltBrakeSw_enum : Outport
  wires:
  UnitConverter/1 -> VHAL_HaltBrakeSw_enum/1
  HaltBrakeSw/1 -> UnitConverter/1

== system halin/HAL_IN/CAN1/EBC1/RmAccelEnSw ==
  RmAccelEnSw : Inport
  UnitConverter : DataTypeConversion  OutDataTypeStr=uint8
  VHAL_RmAccelEnSw_enum : Outport
  wires:
  UnitConverter/1 -> VHAL_RmAccelEnSw_enum/1
  RmAccelEnSw/1 -> UnitConverter/1

== system halin/HAL_IN/CAN1/EBC1/SACtrlBrakeCtrl ==
  SACtrlBrakeCtrl : Inport
  UnitConverter : DataTypeConversion  OutDataTypeStr=uint8
  VHAL_SACtrlBrakeCtrl_SA : Outport
  wires:
  UnitConverter/1 -> VHAL_SACtrlBrakeCtrl_SA/1
  SACtrlBrakeCtrl/1 -> UnitConverter/1

== system halin/HAL_IN/CAN1/EBC1/TractCtrlOvrSw ==
  TractCtrlOvrSw : Inport
  UnitConverter : DataTypeConversion  OutDataTypeStr=uint8
  VHAL_TractCtrlOvrSw_enum : Outport
  wires:
  UnitConverter/1 -> VHAL_TractCtrlOvrSw_enum/1
  TractCtrlOvrSw/1 -> UnitConverter/1

== system halin/HAL_IN/CAN1/EBC1/TrailerABSSta ==
  TrailerABSSta : Inport
  UnitConverter : DataTypeConversion  OutDataTypeStr=uint8
  VHAL_TrailerABSSta_enum : Outport
  wires:
  UnitConverter/1 -> VHAL_TrailerABSSta_enum/1
  TrailerABSSta/1 -> UnitConverter/1

== system halin/HAL_IN/CAN1/EBC1/TrailerABSWarnSig ==
  TrailerABSWarnSig : Inport
  UnitConverter : DataTypeConversion  OutDataTypeStr=uint8
  VHAL_TrailerABSWarnSig_enum : Outport
  wires:
  UnitConverter/1 -> VHAL_TrailerABSWarnSig_enum/1
  TrailerABSWarnSig/1 -> UnitConverter/1

== system halin/HAL_IN/CAN1/EBC2/FASpeed ==
  FASpeed : Inport
  UnitConverter : DataTypeConversion  OutDataTypeStr=uint16
  convert_in : FVT_lib/hal/convert_in  gain=0.0039062  offset=0
  VHAL_FASpeed_kph : Outport
  wires:
  convert_in/1 -> VHAL_FASpeed_kph/1
  UnitConverter/1 -> convert_in/1
  FASpeed/1 -> UnitConverter/1

== system halin/HAL_IN/CAN1/EBC2/RelaSpdFALWheel ==
  RelaSpdFALWheel : Inport
  UnitConverter : DataTypeConversion  OutDataTypeStr=uint8
  convert_in : FVT_lib/hal/convert_in  gain=0.0625  offset=-7.8125
  VHAL_RelaSpdFALWheel_kph : Outport
  wires:
  convert_in/1 -> VHAL_RelaSpdFALWheel_kph/1
  UnitConverter/1 -> convert_in/1
  RelaSpdFALWheel/1 -> UnitConverter/1

== system halin/HAL_IN/CAN1/EBC2/RelaSpdFARWheel ==
  RelaSpdFARWheel : Inport
  UnitConverter : DataTypeConversion  OutDataTypeStr=uint8
  convert_in : FVT_lib/hal/convert_in  gain=0.0625  offset=-7.8125
  VHAL_RelaSpdFARWheel_kph : Outport
  wires:
  convert_in/1 -> VHAL_RelaSpdFARWheel_kph/1
  UnitConverter/1 -> convert_in/1
  RelaSpdFARWheel/1 -> UnitConverter/1

== system halin/HAL_IN/CAN1/EBC5/BrkTempeWarn ==
  BrkTempeWarn : Inport
  UnitConverter : DataTypeConversion  OutDataTypeStr=uint8
  VHAL_BrkTempeWarn_enum : Outport
  wires:
  UnitConverter/1 -> VHAL_BrkTempeWarn_enum/1
  BrkTempeWarn/1 -> UnitConverter/1

== system halin/HAL_IN/CAN1/EBC5/FndBrkUse ==
  FndBrkUse : Inport
  UnitConverter : DataTypeConversion  OutDataTypeStr=uint8
  VHAL_FndBrkUse_enum : Outport
  wires:
  UnitConverter/1 -> VHAL_FndBrkUse_enum/1
  FndBrkUse/1 -> UnitConverter/1

== system halin/HAL_IN/CAN1/EBC5/HaltBrkMode ==
  HaltBrkMode : Inport
  UnitConverter : DataTypeConversion  OutDataTypeStr=uint8
  VHAL_HaltBrkMode_enum : Outport
  wires:
  UnitConverter/1 -> VHAL_HaltBrkMode_enum/1
  HaltBrkMode/1 -> UnitConverter/1

== system halin/HAL_IN/CAN1/EBC5/HillHolderMode ==
  HillHolderMode : Inport
  UnitConverter : DataTypeConversion  OutDataTypeStr=uint8
  VHAL_HillHolderMode_enum : Outport
  wires:
  UnitConverter/1 -> VHAL_HillHolderMode_enum/1
  HillHolderMode/1 -> UnitConverter/1

== system halin/HAL_IN/CAN1/EBC5/ParkBrkActuFAct ==
  ParkBrkActuFAct : Inport
  UnitConverter : DataTypeConversion  OutDataTypeStr=uint8
  VHAL_ParkBrkActuFAct_enum : Outport
  wires:
  UnitConverter/1 -> VHAL_ParkBrkActuFAct_enum/1
  ParkBrkActuFAct/1 -> UnitConverter/1

== system halin/HAL_IN/CAN1/EBC5/XBRAcltnLimit ==
  XBRAcltnLimit : Inport
  UnitConverter : DataTypeConversion  OutDataTypeStr=uint8
  convert_in : FVT_lib/hal/convert_in  gain=0.1  offset=-12.5
  VHAL_XBRAcltnLimit_mps2 : Outport
  wires:
  convert_in/1 -> VHAL_XBRAcltnLimit_mps2/1
  UnitConverter/1 -> convert_in/1
  XBRAcltnLimit/1 -> UnitConverter/1

== system halin/HAL_IN/CAN1/EBC5/XBRActtrlMode ==
  XBRActtrlMode : Inport
  UnitConverter : DataTypeConversion  OutDataTypeStr=uint8
  VHAL_XBRActtrlMode_enum : Outport
  wires:
  UnitConverter/1 -> VHAL_XBRActtrlMode_enum/1
  XBRActtrlMode/1 -> UnitConverter/1

== system halin/HAL_IN/CAN1/EBC5/XBRSysSta ==
  XBRSysSta : Inport
  UnitConverter : DataTypeConversion  OutDataTypeStr=uint8
  VHAL_XBRSysSta_enum : Outport
  wires:
  UnitConverter/1 -> VHAL_XBRSysSta_enum/1
  XBRSysSta/1 -> UnitConverter/1

== system halin/HAL_IN/CAN1/EHPS_Status_1/EHPSEnSta ==
  EHPSEnSta : Inport
  UnitConverter : DataTypeConversion  OutDataTypeStr=uint8
  VHAL_EHPSEnSta_enum : Outport
  wires:
  UnitConverter/1 -> VHAL_EHPSEnSta_enum/1
  EHPSEnSta/1 -> UnitConverter/1

== system halin/HAL_IN/CAN1/EMC1_EM1/EM1CS ==
  EM1CS : Inport
  UnitConverter : DataTypeConversion  OutDataTypeStr=uint8
  VHAL_EM1CS_enum : Outport
  wires:
  UnitConverter/1 -> VHAL_EM1CS_enum/1
  EM1CS/1 -> UnitConverter/1

== system halin/HAL_IN/CAN1/EMC1_EM1/EM1Cnt ==
  EM1Cnt : Inport
  UnitConverter : DataTypeConversion  OutDataTypeStr=uint8
  VHAL_EM1Cnt_enum : Outport
  wires:
  UnitConverter/1 -> VHAL_EM1Cnt_enum/1
  EM1Cnt/1 -> UnitConverter/1

== system halin/HAL_IN/CAN1/EMC1_EM1/EM1OvrCtrlMBrk ==
  EM1OvrCtrlMBrk : Inport
  UnitConverter : DataTypeConversion  OutDataTypeStr=uint8
  VHAL_EM1OvrCtrlMBrk_enum : Outport
  wires:
  UnitConverter/1 -> VHAL_EM1OvrCtrlMBrk_enum/1
  EM1OvrCtrlMBrk/1 -> UnitConverter/1

== system halin/HAL_IN/CAN1/EMC1_EM1/EM1OvrCtrlMDriv ==
  EM1OvrCtrlMDriv : Inport
  UnitConverter : DataTypeConversion  OutDataTypeStr=uint8
  VHAL_EM1OvrCtrlMDriv_enum : Outport
  wires:
  UnitConverter/1 -> VHAL_EM1OvrCtrlMDriv_enum/1
  EM1OvrCtrlMDriv/1 -> UnitConverter/1

== system halin/HAL_IN/CAN1/EMC1_EM1/EM1OvrCtrlMPriBrk ==
  EM1OvrCtrlMPriBrk : Inport
  UnitConverter : DataTypeConversion  OutDataTypeStr=uint8
  VHAL_EM1OvrCtrlMPriBrk_enum : Outport
  wires:
  UnitConverter/1 -> VHAL_EM1OvrCtrlMPriBrk_enum/1
  EM1OvrCtrlMPriBrk/1 -> UnitConverter/1

== system halin/HAL_IN/CAN1/EMC1_EM1/EM1OvrCtrlMPriDriv ==
  EM1OvrCtrlMPriDriv : Inport
  UnitConverter : DataTypeConversion  OutDataTypeStr=uint8
  VHAL_EM1OvrCtrlMPriDriv_enum : Outport
  wires:
  UnitConverter/1 -> VHAL_EM1OvrCtrlMPriDriv_enum/1
  EM1OvrCtrlMPriDriv/1 -> UnitConverter/1

== system halin/HAL_IN/CAN1/EMC1_EM1/EM1ReqTorqHRlsBrk ==
  EM1ReqTorqHRlsBrk : Inport
  UnitConverter : DataTypeConversion  OutDataTypeStr=uint8
  VHAL_EM1ReqTorqHRlsBrk_pct : Outport
  wires:
  UnitConverter/1 -> VHAL_EM1ReqTorqHRlsBrk_pct/1
  EM1ReqTorqHRlsBrk/1 -> UnitConverter/1

== system halin/HAL_IN/CAN1/EMC1_EM1/EM1ReqTorqHRlsDri ==
  EM1ReqTorqHRlsDri : Inport
  UnitConverter : DataTypeConversion  OutDataTypeStr=uint8
  VHAL_EM1ReqTorqHRlsDri_pct : Outport
  wires:
  UnitConverter/1 -> VHAL_EM1ReqTorqHRlsDri_pct/1
  EM1ReqTorqHRlsDri/1 -> UnitConverter/1

== system halin/HAL_IN/CAN1/EMC1_EM1/EM1ReqTorqLimBrk ==
  EM1ReqTorqLimBrk : Inport
  UnitConverter : DataTypeConversion  OutDataTypeStr=uint8
  convert_in : FVT_lib/hal/convert_in  gain=1  offset=-125
  VHAL_EM1ReqTorqLimBrk_pct : Outport
  wires:
  convert_in/1 -> VHAL_EM1ReqTorqLimBrk_pct/1
  UnitConverter/1 -> convert_in/1
  EM1ReqTorqLimBrk/1 -> UnitConverter/1

== system halin/HAL_IN/CAN1/EMC1_EM1/EM1ReqTorqLimDriv ==
  EM1ReqTorqLimDriv : Inport
  UnitConverter : DataTypeConversion  OutDataTypeStr=uint8
  convert_in : FVT_lib/hal/convert_in  gain=1  offset=-125
  VHAL_EM1ReqTorqLimDriv_pct : Outport
  wires:
  convert_in/1 -> VHAL_EM1ReqTorqLimDriv_pct/1
  UnitConverter/1 -> convert_in/1
  EM1ReqTorqLimDriv/1 -> UnitConverter/1

== system halin/HAL_IN/CAN1/EPB1/EPBParkingBrakeSta ==
  EPB_ParkingBrake_Sta : Inport
  UnitConverter : DataTypeConversion  OutDataTypeStr=uint8
  VHAL_EPBParkingBrakeSta_enum : Outport
  wires:
  UnitConverter/1 -> VHAL_EPBParkingBrakeSta_enum/1
  EPB_ParkingBrake_Sta/1 -> UnitConverter/1

== system halin/HAL_IN/CAN1/PDU_Status_1/PDUDCDCRlySta ==
  PDUDCDCRlySta : Inport
  UnitConverter : DataTypeConversion  OutDataTypeStr=uint8
  VHAL_PDUDCDCRlySta_enum : Outport
  wires:
  UnitConverter/1 -> VHAL_PDUDCDCRlySta_enum/1
  PDUDCDCRlySta/1 -> UnitConverter/1

== system halin/HAL_IN/CAN1/PDU_Status_1/PDUEACRlySta ==
  PDUEACRlySta : Inport
  UnitConverter : DataTypeConversion  OutDataTypeStr=uint8
  VHAL_PDUEACRlySta_enum : Outport
  wires:
  UnitConverter/1 -> VHAL_PDUEACRlySta_enum/1
  PDUEACRlySta/1 -> UnitConverter/1

== system halin/HAL_IN/CAN1/PDU_Status_1/PDUEHPSRlySta ==
  PDUEHPSRlySta : Inport
  UnitConverter : DataTypeConversion  OutDataTypeStr=uint8
  VHAL_PDUEHPSRlySta_enum : Outport
  wires:
  UnitConverter/1 -> VHAL_PDUEHPSRlySta_enum/1
  PDUEHPSRlySta/1 -> UnitConverter/1

== system halin/HAL_IN/CAN1/PDU_Status_1/PDUSelfChkSta ==
  PDUSelfChkSta : Inport
  UnitConverter : DataTypeConversion  OutDataTypeStr=uint8
  VHAL_PDUSelfChkSta_enum : Outport
  wires:
  UnitConverter/1 -> VHAL_PDUSelfChkSta_enum/1
  PDUSelfChkSta/1 -> UnitConverter/1

== system halin/HAL_IN/CAN2/IVI1/AmbLighLowBatAlertSW ==
  AmbLigh_LowBatAlert_SW : Inport
  UnitConverter : DataTypeConversion  OutDataTypeStr=uint8
  VHAL_AmbLighLowBatAlertSW_flg : Outport
  wires:
  UnitConverter/1 -> VHAL_AmbLighLowBatAlertSW_flg/1
  AmbLigh_LowBatAlert_SW/1 -> UnitConverter/1

== system halin/HAL_IN/CAN2/IVI1/AmbLighSafetyAlertSW ==
  AmbLigh_SafetyAlert_SW : Inport
  UnitConverter : DataTypeConversion  OutDataTypeStr=uint8
  VHAL_AmbLighSafetyAlertSW_flg : Outport
  wires:
  UnitConverter/1 -> VHAL_AmbLighSafetyAlertSW_flg/1
  AmbLigh_SafetyAlert_SW/1 -> UnitConverter/1

== system halin/HAL_IN/CAN2/IVI1/AmbLightColorSet ==
  AmbLightColorSet : Inport
  UnitConverter : DataTypeConversion  OutDataTypeStr=uint8
  VHAL_AmbLightColorSet_enum : Outport
  wires:
  UnitConverter/1 -> VHAL_AmbLightColorSet_enum/1
  AmbLightColorSet/1 -> UnitConverter/1

== system halin/HAL_IN/CAN2/IVI1/AmbLightDimInDarkSW ==
  AmbLight_DimInDark_SW : Inport
  UnitConverter : DataTypeConversion  OutDataTypeStr=uint8
  VHAL_AmbLightDimInDarkSW_flg : Outport
  wires:
  UnitConverter/1 -> VHAL_AmbLightDimInDarkSW_flg/1
  AmbLight_DimInDark_SW/1 -> UnitConverter/1

== system halin/HAL_IN/CAN2/IVI1/AmbLightSW ==
  AmbLight_SW : Inport
  UnitConverter : DataTypeConversion  OutDataTypeStr=uint8
  VHAL_AmbLightSW_flg : Outport
  wires:
  UnitConverter/1 -> VHAL_AmbLightSW_flg/1
  AmbLight_SW/1 -> UnitConverter/1

== system halin/HAL_IN/CAN2/IVI1/AmbLightWlcmLightSW ==
  AmbLight_WlcmLight_SW : Inport
  UnitConverter : DataTypeConversion  OutDataTypeStr=uint8
  VHAL_AmbLightWlcmLightSW_flg : Outport
  wires:
  UnitConverter/1 -> VHAL_AmbLightWlcmLightSW_flg/1
  AmbLight_WlcmLight_SW/1 -> UnitConverter/1

== system halin/HAL_IN/CAN2/IVI1/FCPFrEvtBtnACMaxReq ==
  FCP_FrEvt_BtnACMaxReq : Inport
  UnitConverter : DataTypeConversion  OutDataTypeStr=uint8
  VHAL_FCPFrEvtBtnACMaxReq_flg : Outport
  wires:
  UnitConverter/1 -> VHAL_FCPFrEvtBtnACMaxReq_flg/1
  FCP_FrEvt_BtnACMaxReq/1 -> UnitConverter/1

== system halin/HAL_IN/CAN2/IVI1/FCPFrEvtBtnACReq ==
  FCP_FrEvt_BtnACReq : Inport
  UnitConverter : DataTypeConversion  OutDataTypeStr=uint8
  VHAL_FCPFrEvtBtnACReq_flg : Outport
  wires:
  UnitConverter/1 -> VHAL_FCPFrEvtBtnACReq_flg/1
  FCP_FrEvt_BtnACReq/1 -> UnitConverter/1

== system halin/HAL_IN/CAN2/IVI1/FCPFrEvtBtnAutoReq ==
  FCP_FrEvt_BtnAutoReq : Inport
  UnitConverter : DataTypeConversion  OutDataTypeStr=uint8
  VHAL_FCPFrEvtBtnAutoReq_flg : Outport
  wires:
  UnitConverter/1 -> VHAL_FCPFrEvtBtnAutoReq_flg/1
  FCP_FrEvt_BtnAutoReq/1 -> UnitConverter/1

== system halin/HAL_IN/CAN2/IVI1/FCPFrEvtBtnSyncReq ==
  FCP_FrEvt_BtnSyncReq : Inport
  UnitConverter : DataTypeConversion  OutDataTypeStr=uint8
  VHAL_FCPFrEvtBtnSyncReq_flg : Outport
  wires:
  UnitConverter/1 -> VHAL_FCPFrEvtBtnSyncReq_flg/1
  FCP_FrEvt_BtnSyncReq/1 -> UnitConverter/1

== system halin/HAL_IN/CAN2/IVI1/IVITimeCheck ==
  IVI_Time_Check : Inport
  UnitConverter : DataTypeConversion  OutDataTypeStr=uint8
  VHAL_IVITimeCheck_enum : Outport
  wires:
  UnitConverter/1 -> VHAL_IVITimeCheck_enum/1
  IVI_Time_Check/1 -> UnitConverter/1

== system halin/HAL_IN/CAN2/IVI1/IVITimeDay ==
  IVI_Time_Day : Inport
  UnitConverter : DataTypeConversion  OutDataTypeStr=uint8
  VHAL_IVITimeDay_DAY : Outport
  wires:
  UnitConverter/1 -> VHAL_IVITimeDay_DAY/1
  IVI_Time_Day/1 -> UnitConverter/1

== system halin/HAL_IN/CAN2/IVI1/IVITimeHour ==
  IVI_Time_Hour : Inport
  UnitConverter : DataTypeConversion  OutDataTypeStr=uint8
  VHAL_IVITimeHour_hr : Outport
  wires:
  UnitConverter/1 -> VHAL_IVITimeHour_hr/1
  IVI_Time_Hour/1 -> UnitConverter/1

== system halin/HAL_IN/CAN2/IVI1/IVITimeMinute ==
  IVI_Time_Minute : Inport
  UnitConverter : DataTypeConversion  OutDataTypeStr=uint8
  VHAL_IVITimeMinute_min : Outport
  wires:
  UnitConverter/1 -> VHAL_IVITimeMinute_min/1
  IVI_Time_Minute/1 -> UnitConverter/1

== system halin/HAL_IN/CAN2/IVI1/IVITimeMonth ==
  IVI_Time_Month : Inport
  UnitConverter : DataTypeConversion  OutDataTypeStr=uint8
  VHAL_IVITimeMonth_MONTH : Outport
  wires:
  UnitConverter/1 -> VHAL_IVITimeMonth_MONTH/1
  IVI_Time_Month/1 -> UnitConverter/1

== system halin/HAL_IN/CAN2/IVI1/IVITimeSecond ==
  IVI_Time_Second : Inport
  UnitConverter : DataTypeConversion  OutDataTypeStr=uint8
  VHAL_IVITimeSecond_s : Outport
  wires:
  UnitConverter/1 -> VHAL_IVITimeSecond_s/1
  IVI_Time_Second/1 -> UnitConverter/1

== system halin/HAL_IN/CAN2/IVI1/IVITimeYear ==
  IVI_Time_Year : Inport
  UnitConverter : DataTypeConversion  OutDataTypeStr=uint8
  convert_in : FVT_lib/hal/convert_in  gain=1  offset=2000
  VHAL_IVITimeYear_YEAR : Outport
  wires:
  convert_in/1 -> VHAL_IVITimeYear_YEAR/1
  UnitConverter/1 -> convert_in/1
  IVI_Time_Year/1 -> UnitConverter/1

== system halin/HAL_IN/CAN2/IVI1/LINKtoDrive ==
  LINKtoDrive : Inport
  UnitConverter : DataTypeConversion  OutDataTypeStr=uint8
  VHAL_LINKtoDrive_flg : Outport
  wires:
  UnitConverter/1 -> VHAL_LINKtoDrive_flg/1
  LINKtoDrive/1 -> UnitConverter/1

== system halin/HAL_IN/CAN2/IVI1/OpenDrOpenWdoSW ==
  OpenDrOpenWdo_SW : Inport
  UnitConverter : DataTypeConversion  OutDataTypeStr=uint8
  VHAL_OpenDrOpenWdoSW_flg : Outport
  wires:
  UnitConverter/1 -> VHAL_OpenDrOpenWdoSW_flg/1
  OpenDrOpenWdo_SW/1 -> UnitConverter/1

== system halin/HAL_IN/CAN2/IVI1/PWCONTINUEUSE ==
  PW_CONTINUE_USE : Inport
  UnitConverter : DataTypeConversion  OutDataTypeStr=uint8
  VHAL_PWCONTINUEUSE_flg : Outport
  wires:
  UnitConverter/1 -> VHAL_PWCONTINUEUSE_flg/1
  PW_CONTINUE_USE/1 -> UnitConverter/1

== system halin/HAL_IN/CAN2/IVI1/SmartEcoModeSW ==
  SmartEco_Mode_SW : Inport
  UnitConverter : DataTypeConversion  OutDataTypeStr=uint8
  VHAL_SmartEcoModeSW_flg : Outport
  wires:
  UnitConverter/1 -> VHAL_SmartEcoModeSW_flg/1
  SmartEco_Mode_SW/1 -> UnitConverter/1

== system halin/HAL_IN/CAN2/IVI2/ACChgCurSet ==
  AC_Chg_Cur_Set : Inport
  UnitConverter : DataTypeConversion  OutDataTypeStr=uint8
  convert_in : FVT_lib/hal/convert_in  gain=1  offset=5
  VHAL_ACChgCurSet_A : Outport
  wires:
  convert_in/1 -> VHAL_ACChgCurSet_A/1
  UnitConverter/1 -> convert_in/1
  AC_Chg_Cur_Set/1 -> UnitConverter/1

== system halin/HAL_IN/CAN2/IVI2/AVMErrSTA ==
  AVM_Err_STA : Inport
  UnitConverter : DataTypeConversion  OutDataTypeStr=uint8
  VHAL_AVMErrSTA_flg : Outport
  wires:
  UnitConverter/1 -> VHAL_AVMErrSTA_flg/1
  AVM_Err_STA/1 -> UnitConverter/1

== system halin/HAL_IN/CAN2/IVI2/AVMOFFRecButt ==
  AVM_OFF_Rec_Butt : Inport
  UnitConverter : DataTypeConversion  OutDataTypeStr=uint8
  VHAL_AVMOFFRecButt_flg : Outport
  wires:
  UnitConverter/1 -> VHAL_AVMOFFRecButt_flg/1
  AVM_OFF_Rec_Butt/1 -> UnitConverter/1

== system halin/HAL_IN/CAN2/IVI2/AVMParkingmode ==
  AVM_Parking_mode : Inport
  UnitConverter : DataTypeConversion  OutDataTypeStr=uint8
  VHAL_AVMParkingmode_enum : Outport
  wires:
  UnitConverter/1 -> VHAL_AVMParkingmode_enum/1
  AVM_Parking_mode/1 -> UnitConverter/1

== system halin/HAL_IN/CAN2/IVI2/AVMparkingcancel ==
  AVM_parking_cancel : Inport
  UnitConverter : DataTypeConversion  OutDataTypeStr=uint8
  VHAL_AVMparkingcancel_enum : Outport
  wires:
  UnitConverter/1 -> VHAL_AVMparkingcancel_enum/1
  AVM_parking_cancel/1 -> UnitConverter/1
